simulink subsystem "RAMsys"  (R2023a)
settings: Solver=VariableStepAuto  StartTime=0.0  StopTime=10.0  RelTol=1e-3
values from neighbouring files (symbols this model uses):
  Ts = 1/(30*rows*cols)    [LDFItest.m]    (also in LDXItest.m; LXFItest.m; LXFXtest.m; LXXItest.m)
libraries: hdlsllib x1
settings Model: Creator=dileepan  LastModifiedBy=dileepan

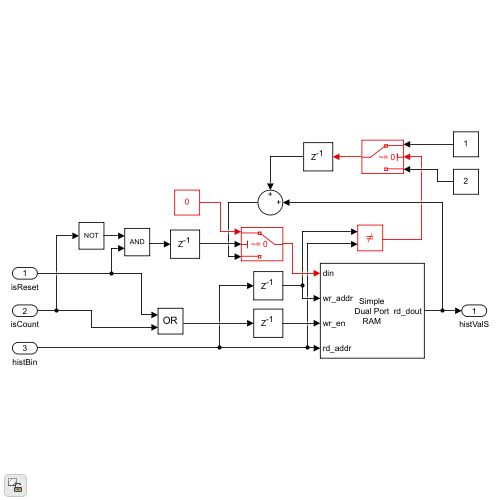
[thumbnail: Simulink's stored preview of the top-level diagram]
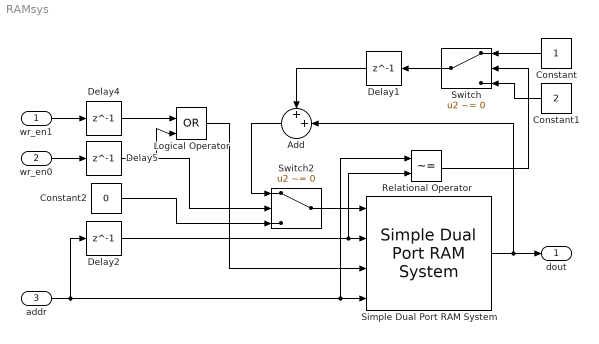
== system RAMsys ==
  wr_en1 : Inport
  wr_en0 : Inport  Port=2
  addr : Inport  Port=3
  Add : Sum  Inputs=++|  AccumDataTypeStr=fixdt(0,ceil(log2(rows*cols)),0)  OutDataTypeStr=Inherit: Same as accumulator
  Constant : Constant  OutDataTypeStr=fixdt(0,2,0)  SampleTime=Ts
  Constant1 : Constant  Value=2  OutDataTypeStr=fixdt(0,2,0)  SampleTime=Ts
  Constant2 : Constant  Value=0  OutDataTypeStr=fixdt(0,ceil(log2(rows*cols)),0)  SampleTime=Ts
  Delay{1..2,4..5} (4 alike) : Delay  DelayLength=1
  Logical Operator : Logic  Operator=OR  IconShape=distinctive  AllPortsSameDT=off  OutDataTypeStr=boolean
  Relational Operator : RelationalOperator  Operator=~=  OutDataTypeStr=boolean  RndMeth=Simplest  InputSameDT=off
  Simple Dual Port RAM System : hdlsllib/HDL RAMs/Simple Dual Port RAM System  RAMType=Simple dual port  WriteOutputValue=New data  RAMInitialValue=0  SimulateUsing=Code generation
  Switch : Switch  Criteria=u2 ~= 0  SaturateOnIntegerOverflow=off  InputSameDT=off
  Switch2 : Switch  Criteria=u2 ~= 0  SaturateOnIntegerOverflow=off  InputSameDT=off
  dout : Outport
  wires:
  Constant1/1 -> Switch/3
  Switch2/1 -> Simple Dual Port RAM System/1
  Constant/1 -> Switch/1
  Delay1/1 -> Add/1
  Switch/1 -> Delay1/1
  Relational Operator/1 -> Switch/2
  Simple Dual Port RAM System/1 -> Add/2, dout/1
  Add/1 -> Switch2/1
  wr_en1/1 -> Delay4/1
  wr_en0/1 -> Delay5/1
  Delay2/1 -> Simple Dual Port RAM System/2, Relational Operator/2
  addr/1 -> Simple Dual Port RAM System/4, Relational Operator/1, Delay2/1
  Delay5/1 -> Switch2/2, Logical Operator/2
  Constant2/1 -> Switch2/3
  Delay4/1 -> Logical Operator/1
  Logical Operator/1 -> Simple Dual Port RAM System/3
